simulink model "Microstick_II_PlusDevBoard_33EP128MC202_ExternalMode_R2015b"  (R2015b)
settings: Solver=FixedStepDiscrete  StartTime=0.0  StopTime=inf  FixedStep=0.01  RelTol=1e-3
undefined symbols (not defined in the file or in its folder): A4, B0, B10, B11, B6, B7, DiscIntNeverNeededParam, Max, ms, P20, P32, P38, P39, P42, P43, Pin, PWMmax, Resol, us
libraries: MCHP_Blockset x13, simulink x1
settings Model: SimulationMode=external  ExtModeTrigDuration=1  Creator=Lubin Kerhuel  LastModifiedBy=M91449
settings DataIOCC: LimitDataPoints=off  SaveFormat=StructureWithTime  SignalLoggingSaveFormat=ModelDataLogs
settings OptimizationCC: OptimizeModelRefInitCode=on  LifeSpan=0.5
settings DebuggingCC: UnderspecifiedInitializationDetection=Classic  MergeDetectMultiDrivingBlocksExec=none  SolverPrmCheckMsg=warning  FcnCallInpInsideContextMsg=EnableAllAsWarning
settings HardwareCC: ProdBitPerInt=16  ProdBitPerPointer=32  ProdLargestAtomicInteger=Integer  ProdLargestAtomicFloat=None  ProdWordSize=16  ProdHWDeviceType=Generic->Custom
settings ModelReferenceCC: ModelReferenceNumInstancesAllowed=Single
settings RTWCC: SystemTargetFile=MCHP_dsPIC_stf.tlc  TemplateMakefile=MCHP_dsPIC.tmf  Description=Microchip Embedded Target PIC24 dsPIC30 dsPIC33 (real-time)  GenerateReport=on  IncludeHyperlinkInReport=on  GenerateTraceInfo=on  GenerateTraceReport=on  GenerateTraceReportSl=on  GenerateTraceReportSf=on  GenerateTraceReportEml=on
settings CodeAppCC: IgnoreCustomStorageClasses=off  MaxIdLength=255  InternalIdentifier=Classic
settings STFCustomTargetCC: TargetLibSuffix=_lib.a  ConcurrentExecutionCompliant=off  IncludeMdlTerminateFcn=off  GeneratePreprocessorConditionals=Use local settings  CombineOutputUpdateFcns=on  ERTCustomFileBanners=on  SupportContinuousTime=off  MATLABClassNameForMDSCustomization=Simulink.SoftwareTarget.ERTCustomization  CPPClassGenCompliant=off  GRTInterface=off  SystemTargetFile=MCHP_dsPIC_stf.tlc
settings ERTTargetCC: TargetLibSuffix=_lib.a  ParMdlRefBuildCompliant=off  CompOptLevelCompliant=off  ConcurrentExecutionCompliant=off  IncludeMdlTerminateFcn=off  ERTFirstTimeCompliant=off  SupportNonInlinedSFcns=on  ModelStepFunctionPrototypeControlCompliant=off  CPPClassGenCompliant=off  UseToolchainInfoCompliant=off  ExtMode=on  ExtModeStaticAlloc=on  ExtModeStaticAllocSize=2048  ExtModeMexFile=ext_serial_win32_comm_no_acks_rtt  ExtModeMexArgs=1 10 115200  ERTSrcFileBannerTemplate=MCHP_dsPIC_code_template.cgt  ERTHdrFileBannerTemplate=MCHP_dsPIC_code_template.cgt  ERTDataSrcFileTemplate=MCHP_dsPIC_code_template.cgt  ERTDataHdrFileTemplate=MCHP_dsPIC_code_template.cgt  ERTCustomFileTemplate=MCHP_main.tlc
settings ConfigComp: CovModelRefEnable=Off

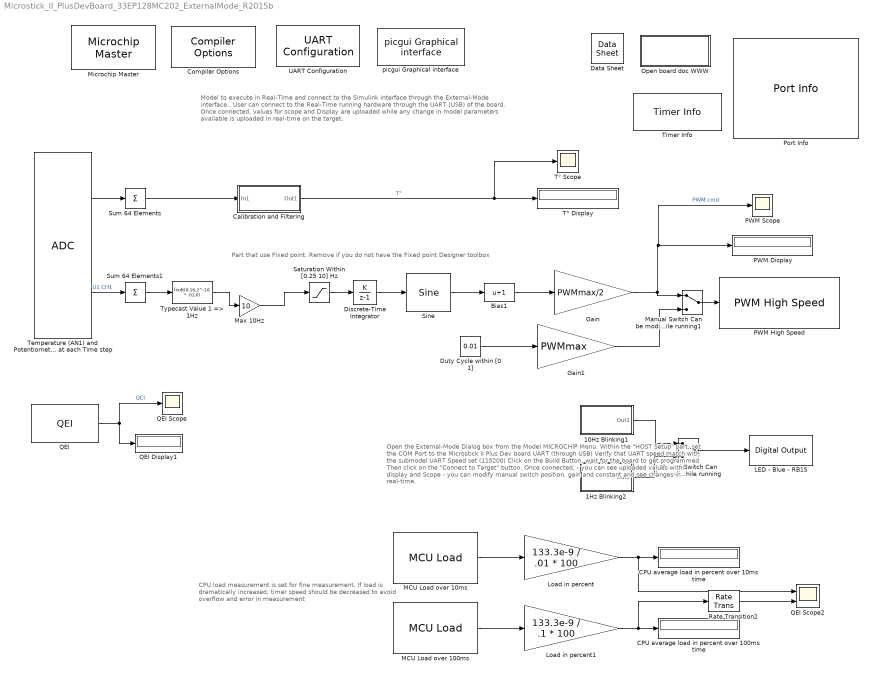
== system Microstick_II_PlusDevBoard_33EP128MC202_ExternalMode_R2015b ==
  note: Model to execute in Real-Time and connect to the Simulink interface through the External-Mode interface..
      | User can connect to the Real-Time running hardware through the UART (USB) of the board.
      | Once connected, values for scope and Display are uploaded
      | while any change in model parameters available is uploaded in real-time on the target.
  note: CPU load measurement is set for fine measurement.
      | If load is dramatically increased, timer speed should
      | be decreased to avoid overflow and error in measurement
  note: Part that use Fixed point. Remove if you do not have the Fixed point Designer toolbox
  note: Open the External-Mode Dialog box from the Model MICROCHIP Menu.
      | Within the "HOST Setup" part, set the COM Port to the Microstick II Plus Dev board UART (through USB)
      | Verify that UART speed match with the submodel UART Speed set (115200)
      | Click on the Build Button, wait for the board to get programmed
      | Then click on the "Connect to Target" button.
      | Once connected,
      | - you can see uploaded values withi display and Scope
      | - you can modify manual switch position, gain and constant and see changes in real-time.
  10Hz Blinking1 : Subsystem
  1Hz Blinking2 : Subsystem
  Bias1 : Bias  Bias=1  SaturateOnIntegerOverflow=on
  CPU average load in percent over 100ms time : Display
  CPU average load in percent over 10ms time : Display
  Calibration and Filtering : Subsystem
  Compiler Options : MCHP_Blockset/System Configuration/Compiler Options  Priority=1  LATEST_CMPLR=on  COMP_LIST=Dynamic Options  COMP_LIST_TXT=xc16 - v1.26  USE_64BIT_DOUBLE=off  MCHP_MULTITHREAD_COMPILATION=on  MCHP_MASTERLINK=Microstick_II_PlusDevBoard_33EP128MC202_ExternalMode_R2015b/Microchip Master  OPTIMIZATION_LEVEL=1  MPLAB_LINKLIB=default  MPLAB_LINKLIB1=default  UNROLL_LOOPS=off  OMIT_FRAME_POINTER=off  PROCEDURAL_ABSTRACTION=off  MCONST=in code memory  MDATA=Can use all available memory  MSCALAR=Can use all available memory  MCODE=is more than 32768  HEAP_SIZE=0  OMF=elf  DEBUG_INFO=off  AssemblyListing=off  ProduceHexOutput=on
  Data Sheet : MCHP_Blockset/System Info/Data Sheet  DOC_Type=datasheet  DOC_MCHP_Id=33FJ64MC802  DOC_FileLastCheckTime=[0 0 0 0 0 0]  cpy_MCHP_Id=33EP128MC202  MCHP_MASTERLINK=Microstick_II_PlusDevBoard_33EP128MC202_ExternalMode_R2015b/Microchip Master
      settings: AttributesFormatString=%<cpy_MCHP_Id>
  Discrete-Time Integrator : DiscreteIntegrator  IntegratorMethod=Accumulation: Forward Euler  gainval=1  InitialConditionSetting=State (most efficient)  SampleTime=.01  OutDataTypeStr=fixdt(0,16,16)  ICPrevOutput=DiscIntNeverNeededParam  ICPrevScaledInput=DiscIntNeverNeededParam
  Duty Cycle within [0 1] : Constant  Value=0.01  OutDataTypeStr=fixdt(0,16,16)
  Gain : Gain  Gain=PWMmax/2  OutDataTypeStr=uint16  RndMeth=Simplest
  Gain1 : Gain  Gain=PWMmax  OutDataTypeStr=uint16  RndMeth=Simplest
  LED - Blue - RB15 : MCHP_Blockset/Digital IO/Digital Output  PORT=Dynamic Options  PORT_TXT="B   [ 0 : 15 ]"  PIN=[15]  PACK=off  SIMULTANEOUS=off  READPREVIOUS=off  ORDERING=None  SampleTime=-1  MCHP_MASTERLINK=Microstick_II_PlusDevBoard_33EP128MC202_ExternalMode_R2015b/Microchip Master
  Load in percent : Gain  Gain=133.3e-9 / .01 * 100  ParamDataTypeStr=Inherit: Inherit from 'Gain'  OutMin=[0]  OutMax=[20]  OutDataTypeStr=single
  Load in percent1 : Gain  Gain=133.3e-9 / .1 * 100  ParamDataTypeStr=Inherit: Inherit from 'Gain'  OutMin=[0]  OutMax=[20]  OutDataTypeStr=single
  MCU Load over 100ms : MCHP_Blockset/Profiling/MCU Load  MCULoadPin=Dynamic Options  MCULoadPin_TXT=None  MCULoadMeasure=on  TIMER_Resolution=Dynamic Options  TIMER_Resolution_TXT="Resol: 0.1333(us)  -  Max: 8.74(ms)"  MCHP_TIMER_REQUEST={MCU_Load}{MCU_Load}21:5:0:0:[]:524288;  MCHP_TIMER_RESULT=[1 65535 ]  MCHP_MASTERLINK=Microstick_II_PlusDevBoard_33EP128MC202_ExternalMode_R2015b/Microchip Master  MCHP_COMPILED_INFO="CompiledSampleTime= [0.10000000000000001   0 ];CompiledInportDataTypes=[ ];CompiledInportDataWidth=[];"  Info="Timer 1:  Resol: 133.304768(ns)  -  Max: 8.73626(ms)"  SampleTime=.1
  MCU Load over 10ms : MCHP_Blockset/Profiling/MCU Load  MCULoadPin=Dynamic Options  MCULoadPin_TXT=None  MCULoadMeasure=on  TIMER_Resolution=Dynamic Options  TIMER_Resolution_TXT="Resol: 0.1333(us)  -  Max: 8.74(ms)"  MCHP_TIMER_REQUEST={MCU_Load}{MCU_Load}21:5:0:0:[]:524288;  MCHP_TIMER_RESULT=[1 65535 ]  MCHP_MASTERLINK=Microstick_II_PlusDevBoard_33EP128MC202_ExternalMode_R2015b/Microchip Master  MCHP_COMPILED_INFO="CompiledSampleTime= [0.01   0 ];CompiledInportDataTypes=[ ];CompiledInportDataWidth=[];"  Info="Timer 1:  Resol: 133.304768(ns)  -  Max: 8.73626(ms)"  SampleTime=.01
  Manual Switch Can be modified while running : ManualSwitch
  Manual Switch Can be modified while running1 : ManualSwitch
  Max 10Hz : Gain  Gain=10  ParamDataTypeStr=fixdt(1,16,8)  OutMin=[0]  OutMax=[20]  OutDataTypeStr=fixdt(0,16)
  Microchip Master : MCHP_Blockset/System Configuration/Microchip Master  Priority=1  PICREF=33EP128MC202  TIMESTEP_REF="ADC  ( 0.01s + [-0.032088%] ==> 0.0099968s )"  BUSYFLAG=Dynamic Options  BUSYFLAG_TXT=None  PWRTEN=PWRT enabled  BOREN=Disable  BODENV=2.7V  BORV=Brown-out Reset set at 2.0V  FPWRT=128ms  DSBOREN=Deep Sleep BOR enabled in Deep Sleep  DSLPBOR=Deep Sleep BOR enabled in Deep Sleep  MCLRE=Enabled  SMCLR=MCLR pin generates a normal system Reset  PMDL1WAY=Allow only one reconfiguration  RSTPRI=Device will obtain reset instruction from Primary flash  TEMP=Not used  SOSCSRC=Analog Mode for use with crystal  SOSCSEL=Secondary oscillator configured for high-power operation  IOL1WAY=Allow multiple reconfigurations  ALTVREF=Voltage reference input; ADC =RA9/RA10 Comparator =RA9;RA10  DISUVREG=Regulator is disabled  DSSWEN=Deep Sleep is controlled by the register bit DSEN  LPCFG=Disabled - regardless of RETEN  RTCBAT=RTC operation is continued through VBAT  VBTBOR=VBAT BOR enabled  WUTSEL=Default regulator start-up time used  POWERSAVE=off  FNOSC=Internal Fast RC (FRC)  FPR=ECIO w/ PLL 16x  FOSFPR=HS3 w/PLL 16x  FOS=Internal Fast RC  FRANGE=High Range  OSCILLATOR_SELECT=Internal Fast RC (FRC)  OSCILLATOR_SELECT_spd=Internal Fast RC (FRC)  QUARTZ=7.37e+06  QUARTZ_spd=7.37e+06  POSCGAIN=2x gain setting  POSCBOOST=Boost the kick start of the oscillator  SOSCGAIN=2x gain setting  SOSCBOOST=Boost the kick start of the oscillator  ACTIV_PLL=on  ACTIV_PLL_spd=on  MIPS_DESIRED=60e6  MIPS_DESIRED_spd=60e6  FPLLMUL=24x Multiplier  FPLLIDIV=8x Divider  POSCFREQ=Primary oscillator/external clock input frequency greater than 8MHz  POSCMD=Primary Oscillator Disabled  POSCMOD=Primary Oscillator Disabled  MIPS=60.012857142857136 * 1e6  FPLLODIV=32x Divider  PLLKEN=Clock switch to PLL source will wait until the PLL lock signal is valid.  FCKSM=Clock switching is enabled;Fail-safe Clock Monitor is disabled  FCKSMEN=Sw Disabled; Mon Disabled  IESO=Start up with FRC; then switch  DSWDTPS=1:2;147;483;648 (25.7 Days)  FWDTEN=Disable  FWDTWINSZ=Window size is 25%  FWPSA=1:512  FWPSA0=1:128  FWPSB=1:16  WDT=Disable  WDTPOST=1:32768  WDTPRE=1:128  WDTPS=1:32768  WINDIS=Watchdog Timer in Non-Window mode  WWDTEN=Non-Window mode  DSWDTEN=DSWDT enabled  DSWDTOSC=DSWDT uses Low Power RC Oscillator (LPRC)  FPBDIV=Pb_Clk is Sys_Clk/8  FSOSCEN=Enable SOSC  LPRCSEL=High Power; High Accuracy Mode  OSCIOFCN=OSCO/CLKO/RA3 functions as CLKO (FOSC/2)  OSCIOFNC=OSC2 is general purpose digital I/O pin  LVRCFG=Low Voltage regulator is not available  PLL_96MHZ=Enabled  PLL96MHZ=96 MHz PLL Startup is enabled automatically on start-up  PLLDIV=PLL is disabled  WDTCLK=WDT uses LPRC  WDTCMX=WDT clock source is determined by the WDTCLK Configuration bits  WDTWIN=WDT Window is 25% of WDT period  APL=Aux Flash Code protect is disabled  APLK=Aux Flash Write Protection or Code Protection is Enabled  AWRP=Aux Flash may be written  BSS=No boot program Flash segment  BWP=Protection Disabled  BWRP=Boot Segment may be written  CP=Protection Disabled  EBS=No Boot EEPROM  ESS=No Segment Data EEPROM  GCP=General Segment Code protect is disabled  GSS=User program memory is not code-protected  GSS0=No protection  GSSK=General Segment Write Protection or Code Protection is Enabled  GWRP=General Segment may be written  PWP=Disable  RBS=No Boot RAM  RSS=No Secure RAM  SSS=No Secure Segment  SWRP=Secure segment may be written  WPCFG=Disable  WPDIS=Disable  WPEND=Write Protect from WPFP to the last page of memory  WPFP=Page 127 (0x1FC00)  ICESEL=Communicate on PGEC1/PGED1  ICS=Communicate on PGEC1 and PGED1  JTAGEN=Disable  COE=Reset Into Operational Mode  RES=Not used  DEBUG=Debugger is disabled  BACKBUG=Not used  BKBUG=Device resets into Operational mode  ALTI2C=I2C mapped to SDA1/SCL1 pins  ALTI2C1=I2C1 mapped to SDA1/SCL1 pins  ALTI2C2=I2C2 mapped to SDA2/SCL2 pins  ALTQIO=QEA1; QEB1; INDX1 are selected as inputs to QEI1  ALTSS1=SS1A is selected as the I/O pin for SPI1  CMPPOL0=Hysteresis is applied to falling edge  CMPPOL1=Hysteresis is applied to falling edge  FCANIO=Default CAN I/O  FETHIO=Default Ethernet I/O  FMIIEN=MII Enabled  FSRSSEL=SRS Priority 7  FUSBIDIO=Controlled by the USB Module  FVBUSONIO=Controlled by USB Module  HPOL=PWM module high side output pins have active-high output polarity  HYST0=45 mV Hysteresis  HYST1=45 mV Hysteresis  I2C1SEL=Use Default SCL1/SDA1 Pins For I2C1  LPOL=PWM module low side output pins have active-high output polarity  PWMPIN=PWM module pins controlled by PORT register at device Reset  RTCOSC=RTCC uses Secondary Oscillator (SOSC)  UPLLEN=USB PLL is enabled  UPLLIDIV=12x Divider  ATMOD8=Not used  ALTPMP=EPMP pins are in default location mode  I2C2SEL=I2C2 is multiplexed to SDA2/RA3 and SCL2/RA2  ALTADREF=AVREF+/AVREF- are mapped to RA9/RA10  ALTCVREF=CVREF+/CVREF- are mapped to RA9/RA10  PWMLOCK=PWM registers may be written without key sequence  MCHP_TIMER_RESULT=[ ]  MCHP_PLLRegisters="[5    226  16387     -1]"  MCHPVAR=MCHP.fcy.periph=MCHP_Fun.Hex2num('[418C9DC9C9249248]');MCHP.fcy.MIPS=MCHP_Fun.Hex2num('[418C9DC9C9249248]');MCHP.PowerSave=0;MCHP.TimeStepFactor=MCHP_Fun.Hex2num('[3FEFFD5F0EEB0E81]');MCHP.TimeStep_Timer=-1;MCHP.NTIMERS=5;MCHP.id.name='33EP128MC202';MCHP.id.N=reshape([33 128 202],1,3);MCHP.id.L=reshape({ 'EP','MC',''},1,3);MCHP.id.Arch=3;MCHP.periph.PPS.reg_RPINRx=reshape([-1 1 1 -1 -1 -1 1 -1 -1 -1 -1 -1 -1 -1 1 1 1 1 -1 -1 -1 -1 -1 -1 1 1 -1 -1 1 1 1 1 -1 -1 -1 -1 1 -1 1 -1 -1 -1 -1 -1 1 1 1 -1 -1 -1 -1 -1 1 -1 -1 -1 -1 -1 -1 -1 -1 -1 -1 -1 -1 -1 -1 -1 -1 -1 -1 -1 -1 -1 -1 1 -1 1 1 1],1,80);MCHP.PPS.dsPIC.RP=reshape([-1 -1 -1 -1 -1 -1 -1 -1 -1 -1 -1 -1 -1 -1 -1 -1 -1 -1 -1 -1 4 -1 -1 -1 -1 -1 -1 -1 -1 -1 -1 -1 -1 -1 -1 19 20 21 22 23 24 25 26 27],1,44);MCHP.PPS.dsPIC.RPI=reshape([-1 -1 -1 -1 -1 -1 -1 -1 -1 -1 -1 -1 -1 -1 -1 -1 -1 -1 -1 -1 -1 -1 -1 -1 -1 -1 -1 -1 -1 -1 -1 -1 16 17 18 -1 -1 -1 -1 -1 -1 -1 -1 -1 28 29 30 31],1,48);MCHP.PPS.dsPIC.RPINR_list=reshape({ '1','INT1','INT2','INT3','INT4','T1CK','T2CK','T3CK','T4CK','T5CK','T6CK','T7CK','T8CK','T9CK','IC1','IC2','IC3','IC4','IC5','IC6','IC7','IC8','OCFA','OCFB','FLT1','FLT2','FLT3','FLT4','QEA1','QEB1','INDX1','HOME1','QEA2','QEB2','INDX2','HOME2','U1RX','U1CTS','U2RX','U2CTS','SDI1','SCK1','SS1','44','SDI2','SCK2','SS2','48','CSDIR','CSCK','COFS','52','C1RX','C2RX','U3RX','U3CTS','U4RX','U4CTS','SDI3','SCK3','SS3','62','SDI4','SCK4','SS4','66','IC9','IC10','IC11','IC12','IC13','IC14','IC15','IC16','OCFC','SYNCI1','SYNCI2','DTCMP1','DTCMP2','DTCMP3','DTCMP4','DTCMP5','DTCMP6','DTCMP7','FLT5','FLT6','FLT7','FLT8','89','SENT1','SENT2','92'},1,92);MCHP.PPS.dsPIC.RPOR_list=reshape({ '1','U1TX','U1RTS','U2TX','U2RTS','SDO1','SCK1','SS1','SDO2','SCK2','SS2','CSDO','CSCK','COFS','C1TX','C2TX','OC1','OC2','OC3','OC4','OC5','OC6','OC7','OC8','C1OUT','C2OUT','C3OUT','U3TX','U3RTS','U4TX','U4RTS','SDO3','SCK3','SS3','SDO4','SCK4','SS4','OC9','OC10','OC11','OC12','OC13','OC14','OC15','OC16','SYNCO1','SYNCO2','QEI1CCMP','QEI2CCMP','REFCLK','C4OUT','C5OUT','52','53','54','55','56','SENT1','SENT2'},1,59);MCHP.PPS.map_RPnR_RPORx=reshape([20 35 36 37 38 39 40 41 42 43],1,10);MCHP.Rx=reshape([2 4 -1 -1 -1 -1 -1 -1 -1 -1 -1 3 5 -1 -1 -1 -1 -1 -1 -1 -1 -1 9 6 -1 -1 -1 -1 -1 -1 -1 -1 -1 10 7 -1 -1 -1 -1 -1 -1 -1 -1 -1 12 11 -1 -1 -1 -1 -1 -1 -1 -1 -1 -1 14 -1 -1 -1 -1 -1 -1 -1 -1 -1 -1 15 -1 -1 -1 -1 -1 -1 -1 -1 -1 -1 16 -1 -1 -1 -1 -1 -1 -1 -1 -1 -1 17 -1 -1 -1 -1 -1 -1 -1 -1 -1 -1 18 -1 -1 -1 -1 -1 -1 -1 -1 -1 -1 21 -1 -1 -1 -1 -1 -1 -1 -1 -1 -1 22 -1 -1 -1 -1 -1 -1 -1 -1 -1 -1 23 -1 -1 -1 -1 -1 -1 -1 -1 -1 -1 24 -1 -1 -1 -1 -1 -1 -1 -1 -1 -1 25 -1 -1 -1 -1 -1 -1 -1 -1 -1 -1 26 -1 -1 -1 -1 -1 -1 -1 -1 -1],11,16);MCHP.ADC.ANtype=reshape([3 0],1,2);MCHP.ADC.ADCONx=reshape([47103 59391 40959 263 0 0],1,6);MCHP.ADC.ADCHS_0=reshape([40863 1799],1,2);MCHP.ADC.Flags=reshape([1 0],1,2);MCHP.ADC.Buffer=reshape([16 -1],1,2);MCHP.ADC.port=reshape([0 1 16 17 18 19 -1 -1 -1 -1 -1 -1 -1 -1 -1 -1 -1 -1 -1 -1 -1 -1 -1 -1 -1 -1 -1 -1 -1 -1 -1 -1 -1 -1 -1 -1 -1 -1 -1 -1 -1 -1 -1 -1 -1 -1 -1 -1 -1 -1 -1 -1 -1 -1 -1 -1 -1],1,57);MCHP.ADC.port_VrefP=17;MCHP.ADC.port_VrefM=16;MCHP.ADC.port_AVdd=-1;MCHP.ADC.port_AVss=-1;MCHP.memory.RAM=16384;MCHP.memory.RAM_XBegin=4096;MCHP.memory.RAM_YBegin=12288;MCHP.memory.RAM_dma=reshape([-1 -1],1,2);MCHP.DMA.Num=4;MCHP.DMA.CNTmax=16383;MCHP.QEI.QEICONx=reshape([49023 -1 -1 -1 -1 -1],1,6);MCHP.QEI.QEItype=1;MCHP.QEI.Port_QEI_INDX=reshape([-1 -1],1,2);MCHP.QEI.Port_QEI_QEA=reshape([-1 -1],1,2);MCHP.QEI.Port_QEI_QEB=reshape([-1 -1],1,2);MCHP.QEI.Port_QEI_UPDN=reshape([-1 -1],1,2);MCHP.INT.Port=reshape([23 32767 32767 -1 -1],1,5);MCHP.PWM_HS.Flags=reshape([3 1 0],1,3);MCHP.PWM.port_FLT=reshape([-1 -1 -1 -1 -1 -1 -1 -1 -1 -1 -1 -1 -1 -1 -1 -1 -1 -1 -1 -1 -1 -1 -1 -1 -1 -1 -1 -1 -1 -1 -1 -1 20],1,33);MCHP.PWM.PWMRef=-1;MCHP.PWM.Flag=0;MCHP.PWM.Port_PWM_l=reshape([31 -1 29 -1 27 -1 -1 -1 -1 -1 -1 -1 -1 -1 -1 -1 -1 -1],2,9);MCHP.PWM.Port_PWM_h=reshape([30 -1 28 -1 26 -1 -1 -1 -1 -1 -1 -1 -1 -1 -1 -1 -1 -1],2,9);MCHP.IC.Port=reshape([32767 32767 32767 32767 0 0 0 0 0 0 0 0 0 0 0 0],1,16);MCHP.IC.type=1;MCHP.OC.Port=reshape([32767 32767 32767 32767 0 0 0 0 0 0 0 0 0 0 0 0],1,16);MCHP.OC.type=1;MCHP.CN.Port=reshape([-1 -1 -1 -1 -1 -1 -1 -1 -1 -1 -1 -1 -1 -1 -1 -1 -1 -1 -1 -1 -1 -1 -1 -1 -1 -1 -1 -1 -1 -1 -1 -1 -1 -1 -1 -1 -1 -1 -1 -1 -1 -1 -1 -1 -1 -1 -1 -1 -1 -1 -1 -1 -1 -1 -1 -1 -1 -1 -1 -1 -1 -1 -1 -1 -1 -1 -1 -1 -1 -1 -1 -1 -1 -1 -1 -1 -1 -1 -1 -1 -1 -1 -1 -1 -1],1,85);MCHP.CN.PullUp=reshape([31 65535 0 0 0 0 0 0 0 0 0],1,11);MCHP.CN.type=1;MCHP.CN.Flag_PullDown=1;MCHP.SPI.Refs=reshape([1 2 0 0 0 0],1,6);MCHP.SPI.SPIxCON1=8191;MCHP.SPI.SPIxCON2=57347;MCHP.SPI.Port_SDI=reshape([25 -1 -1 -1 -1 -1],1,6);MCHP.SPI.Port_SDO=reshape([24 -1 -1 -1 -1 -1],1,6);MCHP.SPI.Port_SCK=reshape([23 -1 -1 -1 -1 -1],1,6);MCHP.SPI.Port_SS=reshape([16 -1 -1 -1 -1 -1],1,6);MCHP.I2C.Refs=reshape([1 2 0 0 0],1,5);MCHP.I2C.I2CxCON=49151;MCHP.I2C.NewRegName=1;MCHP.I2C.Port_SDA=reshape([-1 -1 -1 -1 -1],1,5);MCHP.I2C.Port_SCL=reshape([-1 -1 -1 -1 -1],1,5);MCHP.I2C.Port_ASDA=reshape([25 21 -1 -1 -1],1,5);MCHP.I2C.Port_ASCL=reshape([24 22 -1 -1 -1],1,5);MCHP.I2C.Fuse_Port_SCL_SDA=reshape([3 1 4 1 -1 -1 -1 -1 -1 -1],2,5);MCHP.I2C.Fuse_Port_ASCL_ASDA=reshape([3 2 4 2 -1 -1 -1 -1 -1 -1],2,5);MCHP.Comp.Port_CVrefin=-1;MCHP.Comp.Port_CVref=-1;MCHP.Comp.Port_CVref1O=24;MCHP.Comp.Port_CVref2O=4;MCHP.Comp.Port_CxOUT=reshape([32767 32767 32767 32767 -1],1,5);MCHP.Comp.Port_OAxOUT=reshape([17 0 -1 -1 -1],1,5);MCHP.Comp.Port_CxINP=reshape([18 1 -1 -1 -1],1,5);MCHP.Comp.Port_CxINM=reshape([19 -1 -1 -1 16 -1 -1 -1 -1 -1 -1 -1 -1 -1 -1 -1 -1 -1 -1 -1],4,5);MCHP.Comp.nComp=reshape([4 0 0],1,3);MCHP.Comp.OpAmp=3;MCHP.Comp.CVRCON=reshape([17663 0],1,2);MCHP.UART.port_Rx=reshape([32767 32767 -1 -1 -1 -1],1,6);MCHP.UART.port_Tx=reshape([32767 32767 -1 -1 -1 -1],1,6);MCHP.UART.port_ARx=reshape([-1 -1],1,2);MCHP.UART.port_ATx=reshape([-1 -1],1,2);MCHP.UART.port_RTS=reshape([32767 32767 -1 -1 -1 -1],1,6);MCHP.UART.port_CTS=reshape([32767 32767 -1 -1 -1 -1],1,6);MCHP.UART.reg_UxMODE=reshape([48127 48127 -1 -1 -1 -1],1,6);MCHP.UART.reg_UxSTA=reshape([61439 61439 -1 -1 -1 -1],1,6);  MCHP_CRC=3075413  BTMODE=Device is in Single Boot (legacy) mode  RES1=Not used  PLLSS=PLL is fed by the Primary oscillator  RES2=Not used  ALTCMPI=C1INC is on RB13; C2INC is on RB9 and C3INC is on RA0  BOREN1=BOR Enabled [When BOREN=1]  ALTRB6=Append the RP6/ASCL1/PMPD6 functions of RB6 to RA1 pin functions  RETCFG=Retention regulator is not available  DFMCY=Not used  BSS2=No Boot Segment  BSEN=No Boot Segment  CWRP=Configuration Segment may be written  CSS=No Protection (other than CWRP)  AIVTDIS=Disable Alternate Vector Table  BSLIM=Not used  WDTEN=Disable  BTSWP=Not used  DBCC=Not used  CTXT1=Not Assigned  CTXT2=Not Assigned  SEQNUM=Not used  nSEQNUM=Not used  BOREN0=Enabled  DMTIVT=Not used  DMTCNT=2^31 (2147483648)  DMTEN=Dead Man Timer is Enabled and cannot be disabled by software  ON=Not used  USERID=Not used  RESERVED1=Not used  PGL1WAY=Allow only one reconfiguration  FPLLRNG=34-68 MHz Input  FPLLICLK=FRC is input to the System PLL  FPLLMULT=PLL Multiply by 128  UPLLFSEL=USB PLL input is 24 MHz  DMTINTV=Window/Interval value is 127/128 counter value  WDTSPGM=WDT stops during Flash programming  FDMTEN=Deadman Timer is disabled  TRCEN=Trace features in the CPU are enabled  BOOTISA=Boot code and Exception code is MIPS32  FECCCON=ECC and Dynamic ECC are disabled (ECCCON bits are writable)  EXTDDRSIZE=External DDR2 Size is 128 MB  FSLEEP=Flash is powered down when the device is in Sleep mode  DBGPER=Allow CPU access to all permission regions  EJTAGBEN=Normal EJTAG functionality  TSEQ=Not used  CSEQ=Not used
  Open board doc WWW : Subsystem
      settings: OpenFcn=|
      | web('www.microchip.com/www.microchip.com/en556208','-browser');
      | pause(1);
      | web('www.microchip.com/TCAD0014178791','-browser');
      mask Display: disp('Microstick Plus\nDev Board');
  PWM Display : Display
  PWM High Speed : MCHP_Blockset/PWM IO/PWM High Speed  pop1=[1]  chk1="[0  1  0  0  0]"  chkHL1="[0  1  0  1  1  1  1 ; 0  0  0  1  1  1  1]"  maxP1={ '0.005','0.001','0.001','0.001','0.001','0.001','0.001';'0.001','0.001','1e-06','0.001','0.001','0.001','0.001'}  InitP2={ '0.005','0.001','0.001','0.001','0.001','0.001','0.001';'0.001','0.001','0.001','0.001','0.001','0.001','0.001'}  chkP2="[0  1  0  1  1  1  1 ; 1  0  0  1  1  1  1]"  InitDC={ '0','0','0.0003','50','50','50','50';'0.001','0.001','0.001','50','50','50','50'}  chkDC="[1  1  1  1  1  1  1 ; 0  0  0  1  1  1  1]"  InitPh={ '0','0','0','0.001','0.001','0.001','0.001';'0','0','0','0.001','0.001','0.001','0.001'}  chkPh="[0  0  0  1  1  1  1 ; 0  0  0  1  1  1  1]"  edSEvTrigx={ '0.0001','-1','-1','-1','-1','-1','-1'}  chkSEvTrigx="[0  0  1  1  1  1  1]"  popFlt="[1  1  1  1  1  1  1]"  popFltPin="[24  25  20   4   4   4   4]"  popFltPinRp="[1  1  1  1  1  1  1]"  popFltActivH="[1  2  1  1  1  1  1]"  popFltForceH="[2  2  2  2  2  2  2]"  popFltForceL="[1  1  1  1  1  1  1]"  chkFltBlkOut="[0  0  0  0  0  0  0]"  popDT="[3  3  3  3  3  3  3]"  edDTRx={ '0.02','1e-05','0.001','1e-05','1e-05','1e-05','1e-05'}  edAltDTRx={ '1e-05','0.0001','1e-05','1e-05','1e-05','1e-05','1e-05'}  S_INPUT=[5]  S_INPUT_Size=[1]  S_OUTPUT=[]  S_OUTPUT_Size=[]  S_DWORK_Type=[]  S_DWORK_Size=[]  ADC_VARTRIG={PWM Primary Special Event Trigger;6}  SampleTime=-1  ORDERING=None  MCHP_PORT={PWM2H}{PWM2H}4:4:B12;  MCHP_MASTERLINK=Microstick_II_PlusDevBoard_33EP128MC202_ExternalMode_R2015b/Microchip Master  MCHP_VERSION=v3.38
  PWM Scope : Scope
  Port Info : MCHP_Blockset/System Info/Port Info  MCHP_MASTERLINK=Microstick_II_PlusDevBoard_33EP128MC202_ExternalMode_R2015b/Microchip Master
  QEI : MCHP_Blockset/QEI/QEI  QEI_REF=1  QEI_MODE=Quadrature Encoder  QEI_x2mode=off  QEI_PulseCountDir=Down  PIN_QEA=Dynamic Options  PIN_QEA_TXT=B6 / P38 / Pin[15]  PIN_QEB=Dynamic Options  PIN_QEB_TXT=B7 / P39 / Pin[16]  SWPAB=off  QEAPOL=off  QEBPOL=off  SampleTime=.01  INDXxCNT_Output=is not an output  POSxCNT_Output=is a 16 bits unsigned block output  RESET_Input=off  PIMOD_mode=position is cyclique between user defined boundaries  PIMOD_modeB=Never reset position  PIMOD_reset=on next INDEX event  PIN_INDEX=Dynamic Options  PIN_INDEX_TXT=A4 / P20 / Pin[12]  IMV=QEA = 1 and QEB = 0  IMV_x2=QEA = 1  PIN_HOME=Dynamic Options  PIN_HOME_TXT=A4 / P20 / Pin[12]  QEIxLEC_GEC=[0 256]  QEIxIC=52  PCIIRQ=off  IDXPOL=off  HOMPOL=on  VELxCNT_Output=is not an output  INTxHLD_Output=is not an output  MaxPeriod=1e-3  FILTREN=on  QFDIV_popup=Dynamic Options  QFDIV_popup_TXT=78.14 kHz  FILTER_CutOffFreq=100e3  PIN_CCMP=Dynamic Options  PIN_CCMP_TXT=A4 / P20 / Pin[12]  MCHP_PORT={QEI1 A}{QEA1}5:0:P38;{QEI1 B}{QEB1}5:0:P39;  MCHP_MASTERLINK=Microstick_II_PlusDevBoard_33EP128MC202_ExternalMode_R2015b/Microchip Master  QEI_IntPri=5
  QEI Display1 : Display
  QEI Scope : Scope
  QEI Scope2 : Scope  NumInputPorts=2
  Rate Transition2 : RateTransition  Deterministic=off
  Saturation Within [0.25 10] Hz : Saturate  UpperLimit=10 * .01  LowerLimit=0.25 * .01
  Sine : simulink/Lookup Tables/Sine  Formula=sin(2*pi*u)  NumDataPoints=(2^5)+1  OutputWordLength=16  InternalRulePriority=Speed
  Sum 64 Elements : Sum  Inputs=+
  Sum 64 Elements1 : Sum  Inputs=+
  Temperature (AN1) and Potentiometer (AN0) 64 X 2 Sample&Convert at each Time step : MCHP_Blockset/Analog IO/ADC  Priority=5  ADC_REF=1  Mode=10 bits (allows exact simultaneous sampling)  FORM=0000 dddd dddd dddd ==> Unsigned integer  nSAMPLECHANNELS=CH0 : CH1  nSAMPLECHANNELS_12bits=CH0 only  SIMULTANEOUS=Simultaneously on all Channels  ADxCSS=[1]  MUXA_CH0N=off  MUXA_CH123=Dynamic Options  MUXA_CH123_TXT=AN0 : AN1 : AN2  MUXB_CH0=AN1  MUXB_CH0N=on  MUXB_CH123=Dynamic Options  MUXB_CH123_TXT=AN0 : AN1 : AN2  SequenceRepeat=64  SequenceTiming=are stretcheded to fit exactly previous time step  SSRC_SSRCG=Dynamic Options  SSRC_SSRCG_TXT=6  Update_BlockOutput=After all trig and conversion sequence  Trig_TimeStep=with each update of the ADC block output  ADC_DMA_CHANNEL=use DMA Channel 0  SampleTime=0.01  Info=Total Time for Sample & Conversion : 0.0099968s including 6.9019e-05s (x 64) sample time. Difference with time step is : 3.2088e-06s  MCHP_PORT={Analog Input 0}{AN0}15:2:A0;{Analog Input 1}{AN1}15:2:A1;  MCHP_MASTERLINK=Microstick_II_PlusDevBoard_33EP128MC202_ExternalMode_R2015b/Microchip Master  ADC_TIMING=[0.0099967911637982368]
  Timer Info : MCHP_Blockset/System Info/Timer Info  MCHP_MASTERLINK=Microstick_II_PlusDevBoard_33EP128MC202_ExternalMode_R2015b/Microchip Master
  Typecast Value 1 => 1Hz : DataTypeConversion  OutDataTypeStr=fixdt(0,16,2^-16 * .01,0)  ConvertRealWorld=Stored Integer (SI)
  T° Display : Display
  T° Scope : Scope
  UART Configuration : MCHP_Blockset/BUS UART/UART Configuration  UART_REF=1  BAUD_Choice=Dynamic Options  BAUD_Choice_TXT="115200         [+0.18%]"  BAUD_Choice_IR=Dynamic Options  BAUD_Choice_IR_TXT=[]  BAUD_Custom=115200  IRDA=off  ALT_IO=on  PIN_RX=Dynamic Options  PIN_RX_TXT=B11 / P43 / Pin[22]  PIN_TX=Dynamic Options  PIN_TX_TXT=B10 / P42 / Pin[21]  FlowControl=None  PIN_CTS=Dynamic Options  PIN_CTS_TXT=B0 / P32 / Pin[4]  PIN_RTS=Dynamic Options  PIN_RTS_TXT=A4 / P20 / Pin[12]  MCHP_PORT="{UART1  Rx}{U1RX}3:0:P43;{UART1  Tx}{U1TX}3:1:P42;"  MCHP_MASTERLINK=Microstick_II_PlusDevBoard_33EP128MC202_ExternalMode_R2015b/Microchip Master  MCHP_COM_ExtPil=on  TX_IMPLEMENTATION=Circular Buffer  TX_INT_PRIORITY=5  TX_INT_WHEN=is empty  TX_CIRCULAR_SIZE=128  TX_DMA_CHANNEL="0   (Lowest Priority)"  TX_DMA_SIZE=[]  RX_IMPLEMENTATION=Circular Buffer  RX_INT_PRIORITY=6  RX_INT_WHEN=receive 1 character  RX_CIRCULAR_SIZE=128  InitSequence_chkbox=off  BAUD_Choice_InitSeq=Dynamic Options  BAUD_Choice_InitSeq_TXT="110         [+0.00%]"  BAUD_Choice_IR_InitSeq=Dynamic Options  BAUD_Choice_IR_InitSeq_TXT=0  BAUD_Custom_InitSeq=0  InitSequence='Hello World'
  picgui Graphical interface : MCHP_Blockset/BUS UART/picgui Graphical interface  Nothing=0
  wires:
  Temperature (AN1) and Potentiometer (AN0) 64 X 2 Sample&Convert at each Time step/1 -> Sum 64 Elements/1
  Temperature (AN1) and Potentiometer (AN0) 64 X 2 Sample&Convert at each Time step/2 -> Sum 64 Elements1/1  "U1 CH1"
  Sum 64 Elements/1 -> Calibration and Filtering/1(In1)
  Sum 64 Elements1/1 -> Typecast Value 1 => 1Hz/1
  Manual Switch Can be modified while running/1 -> LED - Blue - RB15/1
  10Hz Blinking1/1(Out1) -> Manual Switch Can be modified while running/1
  1Hz Blinking2/1(Out1) -> Manual Switch Can be modified while running/2
  Calibration and Filtering/1(Out1) -> T° Scope/1, T° Display/1  "T°"
  Sine/1 -> Bias1/1
  Bias1/1 -> Gain/1
  Typecast Value 1 => 1Hz/1 -> Max 10Hz/1
  Discrete-Time Integrator/1 -> Sine/1
  Gain/1 -> PWM Scope/1, PWM Display/1, Manual Switch Can be modified while running1/1  "PWM cmd"
  Max 10Hz/1 -> Saturation Within [0.25 10] Hz/1
  Saturation Within [0.25 10] Hz/1 -> Discrete-Time Integrator/1
  QEI/1 -> QEI Scope/1, QEI Display1/1  "QEI"
  Manual Switch Can be modified while running1/1 -> PWM High Speed/1
  Gain1/1 -> Manual Switch Can be modified while running1/2
  Duty Cycle within [0 1]/1 -> Gain1/1
  MCU Load over 10ms/1 -> Load in percent/1
  Load in percent/1 -> QEI Scope2/1, CPU average load in percent over 10ms time/1
  MCU Load over 100ms/1 -> Load in percent1/1
  Load in percent1/1 -> Rate Transition2/1, CPU average load in percent over 100ms time/1
  Rate Transition2/1 -> QEI Scope2/2

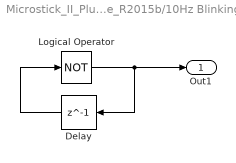
== system Microstick_II_PlusDevBoard_33EP128MC202_ExternalMode_R2015b/10Hz Blinking1 ==
  Delay : Delay  DelayLength=1  InitialCondition=0  InputProcessing=Inherited  SampleTime=.05
  Logical Operator : Logic  Operator=NOT  AllPortsSameDT=off  OutDataTypeStr=boolean
  Out1 : Outport
  wires:
  Logical Operator/1 -> Out1/1, Delay/1
  Delay/1 -> Logical Operator/1

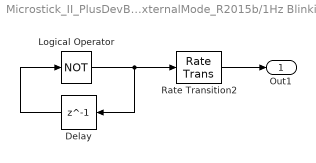
== system Microstick_II_PlusDevBoard_33EP128MC202_ExternalMode_R2015b/1Hz Blinking2 ==
  Delay : Delay  DelayLength=1  InitialCondition=0  InputProcessing=Inherited  SampleTime=.5
  Logical Operator : Logic  Operator=NOT  AllPortsSameDT=off  OutDataTypeStr=boolean
  Rate Transition2 : RateTransition  Deterministic=off  OutPortSampleTime=.05
  Out1 : Outport
  wires:
  Delay/1 -> Logical Operator/1
  Logical Operator/1 -> Delay/1, Rate Transition2/1
  Rate Transition2/1 -> Out1/1

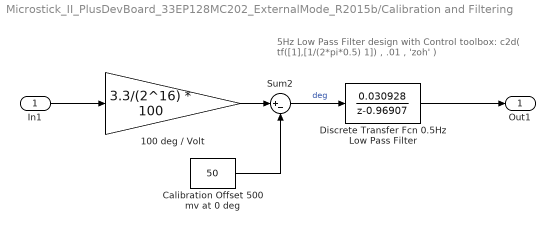
== system Microstick_II_PlusDevBoard_33EP128MC202_ExternalMode_R2015b/Calibration and Filtering ==
  note: 5Hz Low Pass Filter design with Control toolbox:
      | c2d( tf([1],[1/(2*pi*0.5) 1]) , .01 , 'zoh' )
  In1 : Inport
  "100 deg / Volt " : Gain  Gain=3.3/(2^16) * 100  OutDataTypeStr=single
  Calibration Offset 500 mv at 0 deg : Constant  Value=50  OutDataTypeStr=Inherit: Inherit via back propagation  SampleTime=-1
  Discrete Transfer Fcn 0.5Hz Low Pass Filter : DiscreteTransferFcn  Numerator=[0.030928]  Denominator=[1 -0.96907]
  Sum2 : Sum  Inputs=|+-
  Out1 : Outport
  wires:
  Discrete Transfer Fcn 0.5Hz Low Pass Filter/1 -> Out1/1
  In1/1 -> "100 deg / Volt "/1
  "100 deg / Volt "/1 -> Sum2/1
  Calibration Offset 500 mv at 0 deg/1 -> Sum2/2
  Sum2/1 -> Discrete Transfer Fcn 0.5Hz Low Pass Filter/1  "deg"

== system Microstick_II_PlusDevBoard_33EP128MC202_ExternalMode_R2015b/Open board doc WWW ==
